simulink model "matlab2018b"  (R2021a)
settings: Solver=ode4  StartTime=0.0  StopTime=10  FixedStep=0.005  RelTol=1e-3
settings Model: Creator=RIver  LastModifiedBy=xfranklin
settings SolverCC: AlgebraicLoopSolver=TrustRegion
settings DataIOCC: ReturnWorkspaceOutputs=off
settings DebuggingCC: SFMachineParentedDataDiag=warning  ArithmeticOperatorsInVariantConditions=warning
settings SFSimCC: CustomCodeUndefinedFunction=UseInterfaceOnly

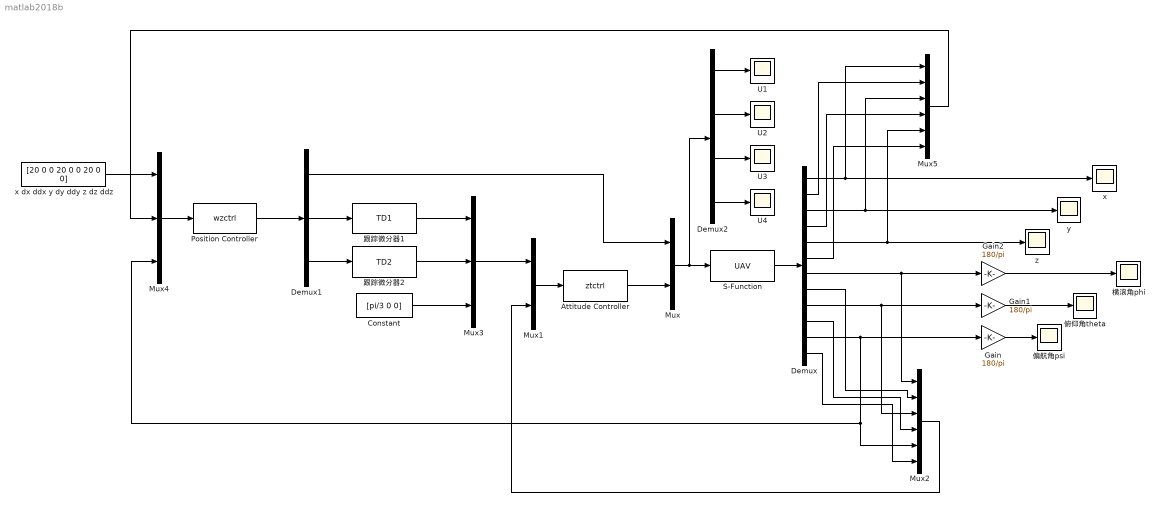
== system matlab2018b ==
  Attitude Controller : S-Function  FunctionName=ztctrl  SFunctionDeploymentMode=off  EnableBusSupport=off
  Constant : Constant  Value=[pi/3 0 0]
  Demux : Demux  Outputs=12
  Demux1 : Demux  Outputs=3
  Demux2 : Demux
  Gain : Gain  Gain=180/pi
  Gain1 : Gain  Gain=180/pi
  Gain2 : Gain  Gain=180/pi
  Mux : Mux  Inputs=2
  Mux1 : Mux  Inputs=2
  Mux2 : Mux  Inputs=6
  Mux3 : Mux  Inputs=3
  Mux4 : Mux  Inputs=3
  Mux5 : Mux  Inputs=6
  Position Controller : S-Function  FunctionName=wzctrl  SFunctionDeploymentMode=off  EnableBusSupport=off
  S-Function : S-Function  FunctionName=UAV  SFunctionDeploymentMode=off  EnableBusSupport=off
  U{1..4} (4 alike) : Scope
  x : Scope
  x dx ddx y dy ddy z dz ddz : Constant  Value=[20 0 0 20 0 0 20 0 0]
  y : Scope
  z : Scope
  俯仰角theta : Scope
  偏航角psi : Scope
  横滚角phi : Scope
  跟踪微分器1 : S-Function  FunctionName=TD1  SFunctionDeploymentMode=off  EnableBusSupport=off
  跟踪微分器2 : S-Function  FunctionName=TD2  SFunctionDeploymentMode=off  EnableBusSupport=off
  wires:
  Mux/1 -> Demux2/1, S-Function/1
  S-Function/1 -> Demux/1
  Demux/3 -> Mux5/3, y/1
  Demux/5 -> Mux5/5, z/1
  Demux/7 -> Mux2/1, Gain2/1
  Demux/9 -> Mux2/3, Gain1/1
  Attitude Controller/1 -> Mux/2
  Mux1/1 -> Attitude Controller/1
  Demux/8 -> Mux2/2
  Demux/10 -> Mux2/4
  Demux/12 -> Mux2/6
  Mux2/1 -> Mux1/2
  Mux3/1 -> Mux1/1
  Constant/1 -> Mux3/3
  跟踪微分器1/1 -> Mux3/1
  跟踪微分器2/1 -> Mux3/2
  Demux1/1 -> Mux/1
  Demux1/2 -> 跟踪微分器1/1
  Demux1/3 -> 跟踪微分器2/1
  Mux5/1 -> Mux4/2
  x dx ddx y dy ddy z dz ddz/1 -> Mux4/1
  Demux/11 -> Mux2/5, Mux4/3, Gain/1
  Position Controller/1 -> Demux1/1
  Mux4/1 -> Position Controller/1
  Demux/2 -> Mux5/2
  Demux/4 -> Mux5/4
  Demux/6 -> Mux5/6
  Demux2/1 -> U1/1
  Demux2/2 -> U2/1
  Demux2/3 -> U3/1
  Demux2/4 -> U4/1
  Gain/1 -> 偏航角psi/1
  Gain1/1 -> 俯仰角theta/1
  Gain2/1 -> 横滚角phi/1
  Demux/1 -> x/1, Mux5/1
